simulink model "FirstCode_Full_CAN_Enable"  (R2014b)
settings: configuration reference "Embedded_Configuration" (kept outside this file)
PreLoadFcn:
  | load('Embedded_Config.mat')
PostLoadFcn:
  | c2000demoscallback(1)
model workspace: external: MAT-File Embedded_Config.mat (data not in the file)
libraries: canmsglib x2, c280xlib x2
settings Model: Creator=The MathWorks Inc.  LastModifiedBy=Nathan

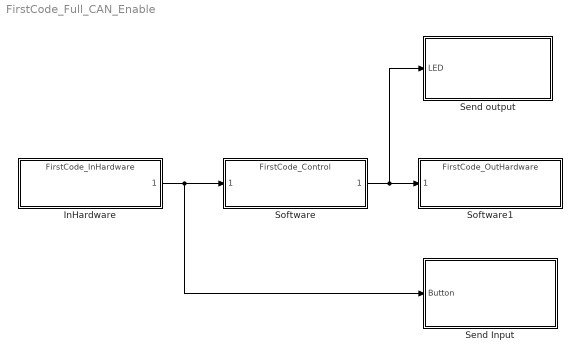
== system FirstCode_Full_CAN_Enable ==
  InHardware : ModelReference  ModelNameDialog=FirstCode_InHardware.slx  SimulationMode=Normal  ModelReferenceVersion=1.90  CopyOfModelName=FirstCode_InHardware.slx  DefaultDataLogging=on
  Send Input : Subsystem
  Send output : Subsystem
  Software : ModelReference  ModelNameDialog=FirstCode_Control.slx  SimulationMode=Normal  ModelReferenceVersion=1.87  CopyOfModelName=FirstCode_Control.slx  DefaultDataLogging=on
  Software1 : ModelReference  ModelNameDialog=FirstCode_OutHardware.slx  SimulationMode=Normal  ModelReferenceVersion=1.87  CopyOfModelName=FirstCode_OutHardware.slx  DefaultDataLogging=on
  wires:
  InHardware/1 -> Send Input/1(Button), Software/1
  Software/1 -> Send output/1(LED), Software1/1

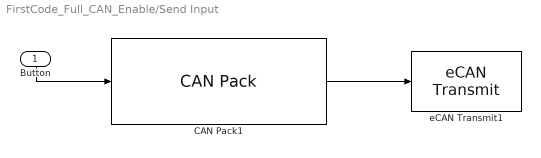
== system FirstCode_Full_CAN_Enable/Send Input ==
  Button : Inport
  CAN Pack1 : canmsglib/CAN Pack  MsgList=(none)  MsgName=Button  MsgIDType=Standard (11-bit identifier)  MsgIdentifier=2  MsgLength=2  SignalInfo=Button$0$16$1$1$1$0$1$0$-Inf$Inf$#  NSignals=1  StartBits=str2num('[int32(0)]')  SignalSizes=str2num('[int32(16)]')  ByteOrders=str2num('[int32(1)]')  DataTypes=str2num('[int32(1)]')  MultiplexTypes=str2num('[int32(1)]')  MultiplexValues=str2num('[double(0)]')  Factors=str2num('[double(1)]')  Offsets=str2num('[double(0)]')  Minimums=str2num('[double(-Inf)]')  Maximums=str2num('[double(Inf)]')  Remote=off
      settings: DataFormat=manually specified signals
  eCAN Transmit1 : c280xlib/eCAN Transmit  chipFamily=C280x  useModule=eCAN_A  mailboxNo=1  messageID=2  messageType=Standard (11-bit identifier)  enableBlockingMode=off  postInterrupt=off  interruptLine=0
  wires:
  Button/1 -> CAN Pack1/1
  CAN Pack1/1 -> eCAN Transmit1/1

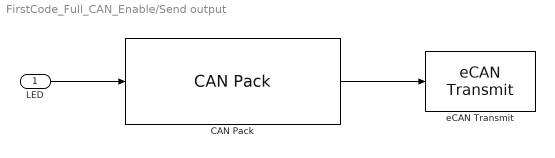
== system FirstCode_Full_CAN_Enable/Send output ==
  LED : Inport
  CAN Pack : canmsglib/CAN Pack  MsgList=(none)  MsgName=LED_Status  MsgIDType=Standard (11-bit identifier)  MsgIdentifier=1  MsgLength=2  SignalInfo=LED$0$16$1$1$1$0$1$0$-Inf$Inf$#  NSignals=1  StartBits=str2num('[int32(0)]')  SignalSizes=str2num('[int32(16)]')  ByteOrders=str2num('[int32(1)]')  DataTypes=str2num('[int32(1)]')  MultiplexTypes=str2num('[int32(1)]')  MultiplexValues=str2num('[double(0)]')  Factors=str2num('[double(1)]')  Offsets=str2num('[double(0)]')  Minimums=str2num('[double(-Inf)]')  Maximums=str2num('[double(Inf)]')  Remote=off
      settings: DataFormat=manually specified signals
  eCAN Transmit : c280xlib/eCAN Transmit  chipFamily=C280x  useModule=eCAN_A  mailboxNo=0  messageID=1  messageType=Standard (11-bit identifier)  enableBlockingMode=off  postInterrupt=off  interruptLine=0
  wires:
  LED/1 -> CAN Pack/1
  CAN Pack/1 -> eCAN Transmit/1
